simulink library "actuators_lib"  (R2018b)
settings: Solver=VariableStepAuto  StartTime=0.0  StopTime=10.0  RelTol=1e-3
undefined symbols (not defined in the file or in its folder): mtq_dipole_body_Am2, mtq_power, mtq_valid, rwa_power, rwa_rpm, rwa_torque_body_Nm, rwa_valid, simParams
libraries: actuator_control_bus x1, actuator_meas_bus x1, mtq_lib x1, reaction_wheel_assembly_lib_disc x1
settings Model: Creator=colem  LastModifiedBy=taylorreynolds

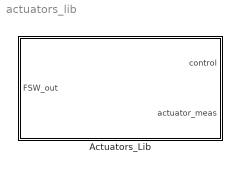
== system actuators_lib ==
  Actuators_Lib : Subsystem

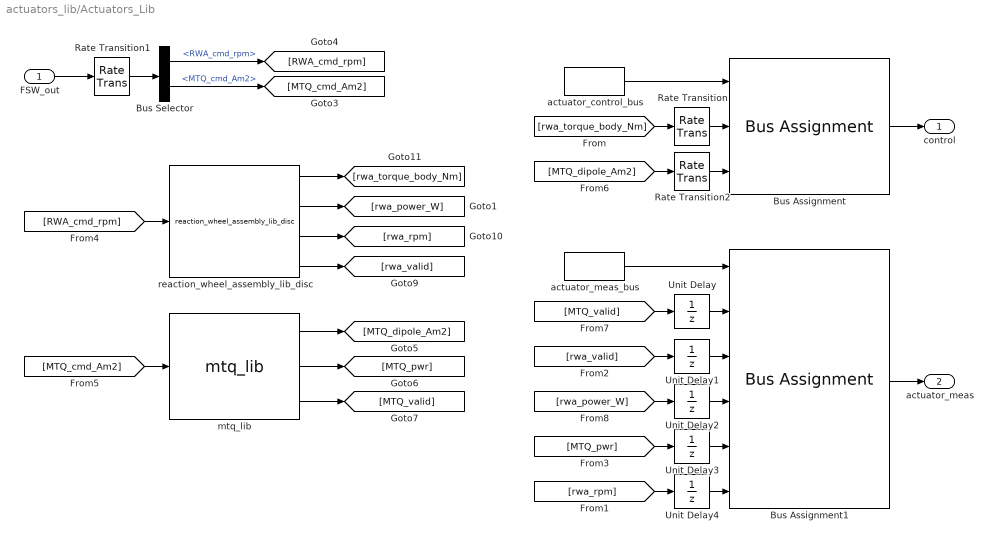
== system actuators_lib/Actuators_Lib ==
  FSW_out : Inport
  Bus Assignment : BusAssignment  AssignedSignals=rwa_torque_body_Nm,mtq_dipole_body_Am2
  Bus Assignment1 : BusAssignment  AssignedSignals=mtq_valid,rwa_valid,rwa_power,mtq_power,rwa_rpm
  Bus Selector : BusSelector  OutputSignals=RWA_cmd_rpm,MTQ_cmd_Am2
  Rate Transition : RateTransition
  Rate Transition1 : RateTransition  OutPortSampleTime=simParams.actuators.sample_time_s
  Rate Transition2 : RateTransition
  Unit Delay : UnitDelay  InitialCondition=true(5,1)  SampleTime=-1
  Unit Delay1 : UnitDelay  InitialCondition=true(4,1)  SampleTime=-1
  Unit Delay2 : UnitDelay  SampleTime=-1
  Unit Delay3 : UnitDelay  SampleTime=-1
  Unit Delay4 : UnitDelay  InitialCondition=simParams.actuators.rwa.ic.rpm  SampleTime=-1
  actuator_control_bus : actuator_control_bus/actuator_control_bus  SystemSampleTime=-1
  actuator_meas_bus : actuator_meas_bus/actuator_meas_bus  SystemSampleTime=-1
  mtq_lib : mtq_lib/mtq_lib  SystemSampleTime=-1
  reaction_wheel_assembly_lib_disc : reaction_wheel_assembly_lib_disc/reaction_wheel_assembly_lib_disc  SystemSampleTime=-1
  control : Outport  OutDataTypeStr=Bus: actuator_control
  actuator_meas : Outport  Port=2  OutDataTypeStr=Bus: actuator_meas
  wires:
  FSW_out/1 -> Rate Transition1/1
  Rate Transition1/1 -> Bus Selector/1
  Bus Selector/2 -> [MTQ_cmd_Am2]  "<MTQ_cmd_Am2>"
  Bus Selector/1 -> [RWA_cmd_rpm]  "<RWA_cmd_rpm>"
  [RWA_cmd_rpm] -> reaction_wheel_assembly_lib_disc/1
  [MTQ_cmd_Am2] -> mtq_lib/1
  mtq_lib/2 -> [MTQ_pwr]
  mtq_lib/1 -> [MTQ_dipole_Am2]
  mtq_lib/3 -> [MTQ_valid]
  reaction_wheel_assembly_lib_disc/3 -> [rwa_rpm]
  reaction_wheel_assembly_lib_disc/2 -> [rwa_power_W]
  reaction_wheel_assembly_lib_disc/1 -> [rwa_torque_body_Nm]
  reaction_wheel_assembly_lib_disc/4 -> [rwa_valid]
  actuator_control_bus/1 -> Bus Assignment/1
  [MTQ_dipole_Am2] -> Rate Transition2/1
  [rwa_torque_body_Nm] -> Rate Transition/1
  Bus Assignment/1 -> control/1
  actuator_meas_bus/1 -> Bus Assignment1/1
  [MTQ_valid] -> Unit Delay/1
  [rwa_valid] -> Unit Delay1/1
  [rwa_power_W] -> Unit Delay2/1
  [MTQ_pwr] -> Unit Delay3/1
  [rwa_rpm] -> Unit Delay4/1
  Bus Assignment1/1 -> actuator_meas/1
  Unit Delay/1 -> Bus Assignment1/2
  Unit Delay1/1 -> Bus Assignment1/3
  Unit Delay2/1 -> Bus Assignment1/4
  Unit Delay3/1 -> Bus Assignment1/5
  Unit Delay4/1 -> Bus Assignment1/6
  Rate Transition/1 -> Bus Assignment/2
  Rate Transition2/1 -> Bus Assignment/3
